simulink model "nn"  (R2023a)
settings: Solver=VariableStepAuto  StartTime=0.0  StopTime=10.0  RelTol=1e-3
libraries: neural x122
(part 1 of 5)
settings Model: Creator=wcheng2014  LastModifiedBy=wcheng2014

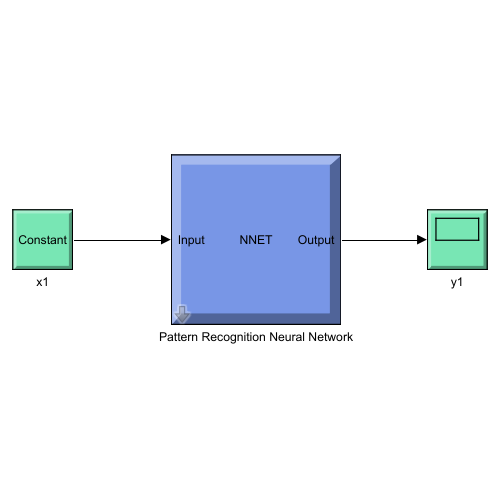
[thumbnail: Simulink's stored preview of the top-level diagram]
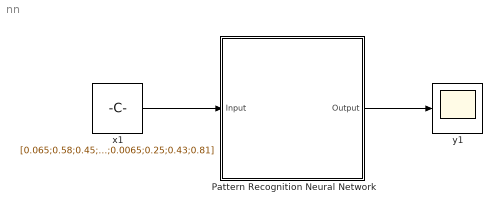
== system nn ==
  Pattern Recognition Neural Network : Subsystem
      mask help: Pattern Recognition Neural Network
      mask Display: e = 0.06;c1 = [120 150 230]/255;c2 = ([120 150 230]+0)/383;c3 = ([120 150 230]+128)/383;patch([0 1 1 0],[0 0 1 1],c1);patch([0 1 1 1-e 1-e 0+e],[0 0 1 1-e 0+e 0+e],c2);patch([0 0 1 1-e 0+e 0+e],[0 1 1 1-e 1-e 0+e],c3);plot([0 1 1 0 0],[0 0 1 1 0]);fprintf('NNET');port_label('input',1,' Input');port_label('output',1,'Output ');
  x1 : Constant  Value=[0.065;0.58;0.45;0.99;0.14;0.69;0.83;0.38;0.61;0.011;0.3;0.76;0.67;0.99;0.5;0.99;0.18;0.81;0.22;0.74;0.0065;0.25;0.43;0.81]  SampleTime=1
      mask Display: e = 0.06;c1 = [120 230 180]/255;c2 = ([120 230 180]+0)/(256+128);c3 = ([120 230 180]+128)/(256+128);patch([0 1 1 0],[0 0 1 1],c1);patch([0 1 1 1-e 1-e 0+e],[0 0 1 1-e 0+e 0+e],c2);patch([0 0 1 1-e 0+e 0+e],[0 1 1 1-e 1-e 0+e],c3);plot([0 1 1 0 0],[0 0 1 1 0]);disp('Constant');
  y1 : Scope
      mask Display: e = 0.06;c1 = [120 230 180]/255;c2 = ([120 230 180]+0)/(256+128);c3 = ([120 230 180]+128)/(256+128);patch([0 1 1 0],[0 0 1 1],c1);patch([0 1 1 1-e 1-e 0+e],[0 0 1 1-e 0+e 0+e],c2);patch([0 0 1 1-e 0+e 0+e],[0 1 1 1-e 1-e 0+e],c3);plot([0 1 1 0 0],[0 0 1 1 0]);plot([0.15 0.85 0.85 0.15 0.15],[0.5 0.5 0.85 0.85 0.5]);
  wires:
  x1/1 -> Pattern Recognition Neural Network/1(Input)
  Pattern Recognition Neural Network/1(Output) -> y1/1

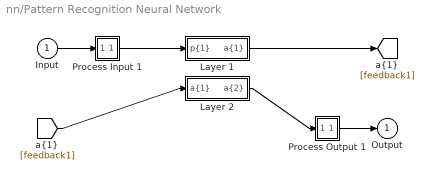
== system nn/Pattern Recognition Neural Network ==
  Input : Inport  PortDimensions=24
      mask Display: e = 0.06;c1 = [120 230 180]/255;c2 = ([120 230 180]+0)/(256+128);c3 = ([120 230 180]+128)/(256+128);patch([0 1 1 0],[0 0 1 1],c1);patch([0 1 1 1-e 1-e 0+e],[0 0 1 1-e 0+e 0+e],c2);patch([0 0 1 1-e 0+e 0+e],[0 1 1 1-e 1-e 0+e],c3);plot([0 1 1 0 0],[0 0 1 1 0]);
  Layer 1 : Subsystem
      mask Display: e = 0.06;c1 = [120 150 230]/255;c2 = ([120 150 230]+0)/383;c3 = ([120 150 230]+128)/383;patch([0 1 1 0],[0 0 1 1],c1);patch([0 1 1 1-e 1-e 0+e],[0 0 1 1-e 0+e 0+e],c2);patch([0 0 1 1-e 0+e 0+e],[0 1 1 1-e 1-e 0+e],c3);plot([0 1 1 0 0],[0 0 1 1 0]);
  Layer 2 : Subsystem
      mask Display: e = 0.06;c1 = [120 150 230]/255;c2 = ([120 150 230]+0)/383;c3 = ([120 150 230]+128)/383;patch([0 1 1 0],[0 0 1 1],c1);patch([0 1 1 1-e 1-e 0+e],[0 0 1 1-e 0+e 0+e],c2);patch([0 0 1 1-e 0+e 0+e],[0 1 1 1-e 1-e 0+e],c3);plot([0 1 1 0 0],[0 0 1 1 0]);
  Process Input 1 : Subsystem
      mask Display: e = 0.06;c1 = [120 150 230]/255;c2 = ([120 150 230]+0)/383;c3 = ([120 150 230]+128)/383;patch([0 1 1 0],[0 0 1 1],c1);patch([0 1 1 1-e 1-e 0+e],[0 0 1 1-e 0+e 0+e],c2);patch([0 0 1 1-e 0+e 0+e],[0 1 1 1-e 1-e 0+e],c3);plot([0 1 1 0 0],[0 0 1 1 0]);
  Process Output 1 : Subsystem
      mask Display: e = 0.06;c1 = [120 150 230]/255;c2 = ([120 150 230]+0)/383;c3 = ([120 150 230]+128)/383;patch([0 1 1 0],[0 0 1 1],c1);patch([0 1 1 1-e 1-e 0+e],[0 0 1 1-e 0+e 0+e],c2);patch([0 0 1 1-e 0+e 0+e],[0 1 1 1-e 1-e 0+e],c3);plot([0 1 1 0 0],[0 0 1 1 0]);
  Output : Outport  InitialOutput=[0;0;0;0;0;0;0;0;0;0;0;0;0;0;0;0;0;0;0]
      mask Display: e = 0.06;c1 = [120 230 180]/255;c2 = ([120 230 180]+0)/(256+128);c3 = ([120 230 180]+128)/(256+128);patch([0 1 1 0],[0 0 1 1],c1);patch([0 1 1 1-e 1-e 0+e],[0 0 1 1-e 0+e 0+e],c2);patch([0 0 1 1-e 0+e 0+e],[0 1 1 1-e 1-e 0+e],c3);plot([0 1 1 0 0],[0 0 1 1 0]);
  wires:
  Input/1 -> Process Input 1/1(x)
  Process Output 1/1(y) -> Output/1
  Process Input 1/1(p) -> Layer 1/1("p{1}")
  Layer 1/1("a{1}") -> [feedback1]
  [feedback1] -> Layer 2/1("a{1} ")
  Layer 2/1("a{2}") -> Process Output 1/1(a)

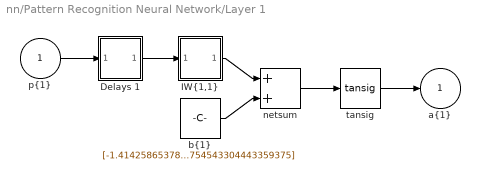
== system nn/Pattern Recognition Neural Network/Layer 1 ==
  "p{1}" : Inport  PortDimensions=24
      mask Display: e = 0.06;c1 = [120 230 180]/255;c2 = ([120 230 180]+0)/(256+128);c3 = ([120 230 180]+128)/(256+128);patch([0 1 1 0],[0 0 1 1],c1);patch([0 1 1 1-e 1-e 0+e],[0 0 1 1-e 0+e 0+e],c2);patch([0 0 1 1-e 0+e 0+e],[0 1 1 1-e 1-e 0+e],c3);plot([0 1 1 0 0],[0 0 1 1 0]);
  Delays 1 : Subsystem
      mask Display: e = 0.06;c1 = [120 150 230]/255;c2 = ([120 150 230]+0)/383;c3 = ([120 150 230]+128)/383;patch([0 1 1 0],[0 0 1 1],c1);patch([0 1 1 1-e 1-e 0+e],[0 0 1 1-e 0+e 0+e],c2);patch([0 0 1 1-e 0+e 0+e],[0 1 1 1-e 1-e 0+e],c3);plot([0 1 1 0 0],[0 0 1 1 0]);disp('0');
  "IW{1,1}" : Subsystem
      mask Display: e = 0.06;c1 = [120 150 230]/255;c2 = ([120 150 230]+0)/383;c3 = ([120 150 230]+128)/383;patch([0 1 1 0],[0 0 1 1],c1);patch([0 1 1 1-e 1-e 0+e],[0 0 1 1-e 0+e 0+e],c2);patch([0 0 1 1-e 0+e 0+e],[0 1 1 1-e 1-e 0+e],c3);plot([0 1 1 0 0],[0 0 1 1 0]);disp('W');
  "b{1}" : Constant  Value=[-1.4142586537889361153474965249188244342803955078125;-1.1695644614589537635396254700026474893093109130859375;1.67760629524994886452304854174144566059112548828125;1.4277868394710127031288493526517413556575775146484375;1.2985162391085343092100856665638275444507598876953125;-1.2621595997541283917797727553988806903362274169921875;-1.5297487787980788009889465683954767882823944091796875;-1.5293583197340769874728039212641306221485137939453125;0.6776465319515077023737603667541407048702239990234375;-0.93538177220409723933158829822787083685398101806640625;-1.277535889187028761426745404605753719806671142578125;1.1029058677491792028746431242325343191623687744140625;0.95217229152203930464537506850319914519786834716796875;1.0352537776093557742029815926798619329929351806640625;-1.340899260898384515172665487625636160373687744140625;0.93659855475700892757373594577074982225894927978515625;-1.1524672792419445865874649825855158269405364990234375;0.74857957572343825081162549395230598747730255126953125;-1.182516750542461192452492468873970210552215576171875;0.72428624181148404392871498203021474182605743408203125;-0.82285027069276939215569655061699450016021728515625;-0.56728469732308273165699574747122824192047119140625;-0.89635793830185328534554400903289206326007843017578125;-0.7465280741878899117835999277303926646709442138671875;-0.83971547546758273927736127006937749683856964111328125;0.7317557191767540825111382218892686069011688232421875;0.84860002552919888696436601094319485127925872802734375;0.62527262099536928818821479580947197973728179931640625;-0.60637075565120224229787027070415206253528594970703125;0.62961571470170418773903975306893698871135711669921875;-0.35989909278169085471432708800421096384525299072265625;0.374207145547579445032937428550212644040584564208984375;-0.58277037487829963513519260231987573206424713134765625;0.19942119566341520719987556731211952865123748779296875;0.449668993385554827124650500991265289485454559326171875;0.271922846350390212677439194521866738796234130859375;-0.50005277717758322975072360350168310105800628662109375;0.204655991022005434576414018010837025940418243408203125;0.75216933771036342815108355353004299104213714599609375;-0.129173697734639991718808005316532216966152191162109375;-0.23580233831504349151231281211948953568935394287109375;-0.32843087962146577662991830948158167302608489990234375;-0.07223232070631192824894384330036700703203678131103515625;0.32637383281239340515611502269166521728038787841796875;-0.40562787064387950675126148780691437423229217529296875;0.15873746850755876547367506645969115197658538818359375;0.1049832060904107022825115791420103050768375396728515625;-0.0181321585518762103117484940639769774861633777618408203125;-0.10584460786044648517023603062625625170767307281494140625;0.0042473883480905645637637491063287598080933094024658203125;0.195890186278736389002830264871590770781040191650390625;0.0480009323559285328020251881753210909664630889892578125;0.370825922311421363186667576883337460458278656005859375;-0.2010369446057873599187360014184378087520599365234375;0.1765263213480416648604176543813082389533519744873046875;-0.173348850511180374578401597318588756024837493896484375;-0.436991329930836502892788075769203715026378631591796875;-0.34230850366641885074159290525130927562713623046875;0.0717400483325078830443288779861177317798137664794921875;0.2474272694052397636443885176049661822617053985595703125;-0.50698425198559193827207991489558480679988861083984375;0.0977340964546310753124913617284619249403476715087890625;-0.428962561510694062594239994723466224968433380126953125;0.51073286420469632407304061416652984917163848876953125;-0.64704721644684182191298305042437277734279632568359375;0.49248779210736082223576204341952688992023468017578125;0.281921517140315491811719539327896200120449066162109375;0.61114075386009714119239788487902842462062835693359375;-0.58884431443021600927067993325181305408477783203125;-0.426517179771635557283815387563663534820079803466796875 ...(+1644 chars)]
      mask Display: e = 0.06;c1 = [120 150 230]/255;c2 = ([120 150 230]+0)/383;c3 = ([120 150 230]+128)/383;patch([0 1 1 0],[0 0 1 1],c1);patch([0 1 1 1-e 1-e 0+e],[0 0 1 1-e 0+e 0+e],c2);patch([0 0 1 1-e 0+e 0+e],[0 1 1 1-e 1-e 0+e],c3);plot([0 1 1 0 0],[0 0 1 1 0]);disp('b');
  netsum : Sum  Inputs=2  InputSameDT=on  SaturateOnIntegerOverflow=on  OutDataTypeStr=Inherit: Same as first input
      mask Display: e = 0.06;c1 = [120 150 230]/255;c2 = ([120 150 230]+0)/383;c3 = ([120 150 230]+128)/383;patch([0 1 1 0],[0 0 1 1],c1);patch([0 1 1 1-e 1-e 0+e],[0 0 1 1-e 0+e 0+e],c2);patch([0 0 1 1-e 0+e 0+e],[0 1 1 1-e 1-e 0+e],c3);plot([0 1 1 0 0],[0 0 1 1 0]);disp('+');
  tansig : neural/Transfer Functions/tansig
  "a{1}" : Outport  InitialOutput=[0;0;0;0;0;0;0;0;0;0;0;0;0;0;0;0;0;0;0;0;0;0;0;0;0;0;0;0;0;0;0;0;0;0;0;0;0;0;0;0;0;0;0;0;0;0;0;0;0;0;0;0;0;0;0;0;0;0;0;0;0;0;0;0;0;0;0;0;0;0;0;0;0;0;0;0;0;0;0;0;0;0;0;0;0;0;0;0;0;0;0;0;0;0;0;0;0;0;0;0]
      mask Display: e = 0.06;c1 = [120 230 180]/255;c2 = ([120 230 180]+0)/(256+128);c3 = ([120 230 180]+128)/(256+128);patch([0 1 1 0],[0 0 1 1],c1);patch([0 1 1 1-e 1-e 0+e],[0 0 1 1-e 0+e 0+e],c2);patch([0 0 1 1-e 0+e 0+e],[0 1 1 1-e 1-e 0+e],c3);plot([0 1 1 0 0],[0 0 1 1 0]);
  wires:
  "p{1}"/1 -> Delays 1/1("p{1}")
  Delays 1/1("pd{1,1}") -> "IW{1,1}"/1("pd{1,1}")
  "IW{1,1}"/1("iz{1,1}") -> netsum/1
  "b{1}"/1 -> netsum/2
  netsum/1 -> tansig/1
  tansig/1 -> "a{1}"/1

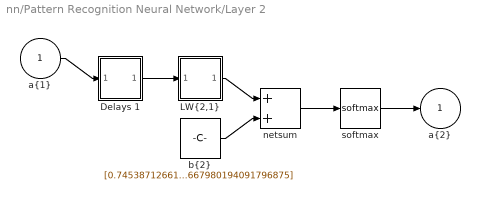
== system nn/Pattern Recognition Neural Network/Layer 2 ==
  "a{1} " : Inport  PortDimensions=100
      mask Display: e = 0.06;c1 = [120 230 180]/255;c2 = ([120 230 180]+0)/(256+128);c3 = ([120 230 180]+128)/(256+128);patch([0 1 1 0],[0 0 1 1],c1);patch([0 1 1 1-e 1-e 0+e],[0 0 1 1-e 0+e 0+e],c2);patch([0 0 1 1-e 0+e 0+e],[0 1 1 1-e 1-e 0+e],c3);plot([0 1 1 0 0],[0 0 1 1 0]);
  Delays 1 : Subsystem
      mask Display: e = 0.06;c1 = [120 150 230]/255;c2 = ([120 150 230]+0)/383;c3 = ([120 150 230]+128)/383;patch([0 1 1 0],[0 0 1 1],c1);patch([0 1 1 1-e 1-e 0+e],[0 0 1 1-e 0+e 0+e],c2);patch([0 0 1 1-e 0+e 0+e],[0 1 1 1-e 1-e 0+e],c3);plot([0 1 1 0 0],[0 0 1 1 0]);disp('0');
  "LW{2,1}" : Subsystem
      mask Display: e = 0.06;c1 = [120 150 230]/255;c2 = ([120 150 230]+0)/383;c3 = ([120 150 230]+128)/383;patch([0 1 1 0],[0 0 1 1],c1);patch([0 1 1 1-e 1-e 0+e],[0 0 1 1-e 0+e 0+e],c2);patch([0 0 1 1-e 0+e 0+e],[0 1 1 1-e 1-e 0+e],c3);plot([0 1 1 0 0],[0 0 1 1 0]);disp('W');
  "b{2}" : Constant  Value=[0.74538712661551576044161038225865922868251800537109375;-0.69394996950398979418395128959673456847667694091796875;0.0190592200685446334917916288986816653050482273101806640625;-0.0976722126513131227998343319995910860598087310791015625;0.69382300776607219727765141215058974921703338623046875;0.325028072645112964256242094052140600979328155517578125;1.04912695954516355101304725394584238529205322265625;0.2108335366438205127348481937588076107203960418701171875;0.67349340234099275281920427005388773977756500244140625;0.007548940634630994968301553882383814197964966297149658203125;-0.016552177459163548711718050299168680794537067413330078125;-0.67800700649082135118561609488097019493579864501953125;0.215769854572676889059579252716503106057643890380859375;0.814351602218465142613013085792772471904754638671875;-0.047890675980428232261232324162847362458705902099609375;0.0588166109055049124432201779200113378465175628662109375;0.49057526188050359916559273187885992228984832763671875;-0.75367055023117668355325804441235959529876708984375;0.73513818780673989561336156839388422667980194091796875]
      mask Display: e = 0.06;c1 = [120 150 230]/255;c2 = ([120 150 230]+0)/383;c3 = ([120 150 230]+128)/383;patch([0 1 1 0],[0 0 1 1],c1);patch([0 1 1 1-e 1-e 0+e],[0 0 1 1-e 0+e 0+e],c2);patch([0 0 1 1-e 0+e 0+e],[0 1 1 1-e 1-e 0+e],c3);plot([0 1 1 0 0],[0 0 1 1 0]);disp('b');
  netsum : Sum  Inputs=2  InputSameDT=on  SaturateOnIntegerOverflow=on  OutDataTypeStr=Inherit: Same as first input
      mask Display: e = 0.06;c1 = [120 150 230]/255;c2 = ([120 150 230]+0)/383;c3 = ([120 150 230]+128)/383;patch([0 1 1 0],[0 0 1 1],c1);patch([0 1 1 1-e 1-e 0+e],[0 0 1 1-e 0+e 0+e],c2);patch([0 0 1 1-e 0+e 0+e],[0 1 1 1-e 1-e 0+e],c3);plot([0 1 1 0 0],[0 0 1 1 0]);disp('+');
  softmax : neural/Transfer Functions/softmax
  "a{2}" : Outport  InitialOutput=[0;0;0;0;0;0;0;0;0;0;0;0;0;0;0;0;0;0;0]
      mask Display: e = 0.06;c1 = [120 230 180]/255;c2 = ([120 230 180]+0)/(256+128);c3 = ([120 230 180]+128)/(256+128);patch([0 1 1 0],[0 0 1 1],c1);patch([0 1 1 1-e 1-e 0+e],[0 0 1 1-e 0+e 0+e],c2);patch([0 0 1 1-e 0+e 0+e],[0 1 1 1-e 1-e 0+e],c3);plot([0 1 1 0 0],[0 0 1 1 0]);
  wires:
  "a{1} "/1 -> Delays 1/1("p{2}")
  Delays 1/1("pd{2,1}") -> "LW{2,1}"/1("ad{2,1}")
  "LW{2,1}"/1("lz{2,1}") -> netsum/1
  "b{2}"/1 -> netsum/2
  netsum/1 -> softmax/1
  softmax/1 -> "a{2}"/1

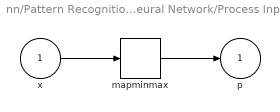
== system nn/Pattern Recognition Neural Network/Process Input 1 ==
  x : Inport  PortDimensions=24
      mask Display: e = 0.06;c1 = [120 230 180]/255;c2 = ([120 230 180]+0)/(256+128);c3 = ([120 230 180]+128)/(256+128);patch([0 1 1 0],[0 0 1 1],c1);patch([0 1 1 1-e 1-e 0+e],[0 0 1 1-e 0+e 0+e],c2);patch([0 0 1 1-e 0+e 0+e],[0 1 1 1-e 1-e 0+e],c3);plot([0 1 1 0 0],[0 0 1 1 0]);
  mapminmax : neural/Processing Functions/mapminmax  xmin=[-0.00936862991662801292136464326177;-0.00752766203843835413067608897109;-0.00581546906331542601265027769841;-0.00163195697078499790677597047761;-0.00161192041666335938998599885963;-0.00199194405856983891567324462812;-0.00239743942073822324800858041272;-0.00165927896889872528163323295303;-0.00462083476200803033862030133605;-0.000589138937315603072875092038885;-0.00342971649845846826565320952795;-0.00178829204643937700325295736548;-0.000294164325540524629332139738835;-0.00510630338254758342486638866831;-0.00433054445966396528433506318834;-0.00173365368762512517264440248255;-0.00209873568298757362526885117404;-0.0021232461186304618649955955334;-0.00393684503808566788052303309087;-0.00354362846861056013381130469497;-0.00224125120222895546362451568712;-0.000883853421884683854159447946586;-0.00279873140063191527815433801152;-0.000979416489782725108170780004002]  xmax=[0.0251902612616419219193630851805;0.0156063317468424500589208037127;0.016482558063239505230512804701;0.016741573775329587903115680092;0.0112162936322919293274935625959;0.00846873685133964215765445260331;0.00566374315210627088390538119711;0.00797428414978496036269461910706;0.00810518675162219537355667853262;0.00530159547171926703867939068004;0.0050255271308770055327386216959;0.00726227156441705545830700430088;0.00689363124012842831689340528101;0.0039974047177082638881984166801;0.00465776629890068960548887844197;0.00407681169784757102547700924333;0.00292020531382863879343858570792;0.00507241104868061398747158818878;0.0063662824889485492008134315256;0.00572535644046823222197417635471;0.00207216685717126480881233874243;0.00674146165124112073385731491726;0.00824949744851899424702423857525;0.00353990445699725597705764812417]  ymin=-1  ymax=1
  p : Outport  PortDimensions=24
      mask Display: e = 0.06;c1 = [120 230 180]/255;c2 = ([120 230 180]+0)/(256+128);c3 = ([120 230 180]+128)/(256+128);patch([0 1 1 0],[0 0 1 1],c1);patch([0 1 1 1-e 1-e 0+e],[0 0 1 1-e 0+e 0+e],c2);patch([0 0 1 1-e 0+e 0+e],[0 1 1 1-e 1-e 0+e],c3);plot([0 1 1 0 0],[0 0 1 1 0]);
  wires:
  x/1 -> mapminmax/1
  mapminmax/1 -> p/1

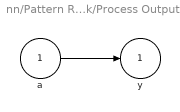
== system nn/Pattern Recognition Neural Network/Process Output 1 ==
  a : Inport  PortDimensions=19
      mask Display: e = 0.06;c1 = [120 230 180]/255;c2 = ([120 230 180]+0)/(256+128);c3 = ([120 230 180]+128)/(256+128);patch([0 1 1 0],[0 0 1 1],c1);patch([0 1 1 1-e 1-e 0+e],[0 0 1 1-e 0+e 0+e],c2);patch([0 0 1 1-e 0+e 0+e],[0 1 1 1-e 1-e 0+e],c3);plot([0 1 1 0 0],[0 0 1 1 0]);
  y : Outport  PortDimensions=19
      mask Display: e = 0.06;c1 = [120 230 180]/255;c2 = ([120 230 180]+0)/(256+128);c3 = ([120 230 180]+128)/(256+128);patch([0 1 1 0],[0 0 1 1],c1);patch([0 1 1 1-e 1-e 0+e],[0 0 1 1-e 0+e 0+e],c2);patch([0 0 1 1-e 0+e 0+e],[0 1 1 1-e 1-e 0+e],c3);plot([0 1 1 0 0],[0 0 1 1 0]);
  wires:
  a/1 -> y/1

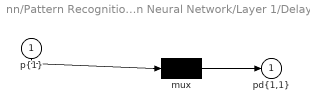
== system nn/Pattern Recognition Neural Network/Layer 1/Delays 1 ==
  "p{1}" : Inport  PortDimensions=24
      mask Display: e = 0.06;c1 = [120 230 180]/255;c2 = ([120 230 180]+0)/(256+128);c3 = ([120 230 180]+128)/(256+128);patch([0 1 1 0],[0 0 1 1],c1);patch([0 1 1 1-e 1-e 0+e],[0 0 1 1-e 0+e 0+e],c2);patch([0 0 1 1-e 0+e 0+e],[0 1 1 1-e 1-e 0+e],c3);plot([0 1 1 0 0],[0 0 1 1 0]);
  mux : Mux  Inputs=1
      mask Display: e = 0.06;c1 = [120 150 230]/255;c2 = ([120 150 230]+0)/383;c3 = ([120 150 230]+128)/383;patch([0 1 1 0],[0 0 1 1],c1);patch([0 1 1 1-e 1-e 0+e],[0 0 1 1-e 0+e 0+e],c2);patch([0 0 1 1-e 0+e 0+e],[0 1 1 1-e 1-e 0+e],c3);plot([0 1 1 0 0],[0 0 1 1 0]);disp('Mux')
  "pd{1,1}" : Outport
      mask Display: e = 0.06;c1 = [120 230 180]/255;c2 = ([120 230 180]+0)/(256+128);c3 = ([120 230 180]+128)/(256+128);patch([0 1 1 0],[0 0 1 1],c1);patch([0 1 1 1-e 1-e 0+e],[0 0 1 1-e 0+e 0+e],c2);patch([0 0 1 1-e 0+e 0+e],[0 1 1 1-e 1-e 0+e],c3);plot([0 1 1 0 0],[0 0 1 1 0]);
  wires:
  "p{1}"/1 -> mux/1
  mux/1 -> "pd{1,1}"/1
